simulink model "VELO1"  (R2019b)
settings: Solver=FixedStepAuto  StartTime=0.0  StopTime=t(end)  FixedStep=0.01  RelTol=1e-3
libraries: eeGeneralControl x26, dspstat3 x15, dspfdesign x11, sharedTrackingLibrary x2
(part 2 of 2)

== matlab function VELO1/Raw data filer /Subsystem2/MATLAB Function ==
  data: z1 input; x_hat output; z2 input; z3 input
function x_hat=fusion(z1,z2,z3)
% Kalman Filter sensor fusion example based on
%  
% http://www.slideshare.net/antoniomorancardenas/data-fusion-with-kalman-filtering
%
% % See http://home.wlu.edu/~levys/kalman_tutorial for background

% Copyright (C) 2014 Simon D. Levy
%
% This code is free software: you can redistribute it and/or modify
% it under the terms of the GNU Lesser General Public License as
% published by the Free Software Foundation, either version 3 of the
% License, or (at your option) any later version.
%
% This code is distributed in the hope that it will be useful,
% but WITHOUT ANY WARRANTY without even the implied warranty of
% MERCHANTABILITY or FITNESS FOR A PARTICULAR PURPOSE. See the
% GNU General Public License for more details.
%
% You should have received a copy of the GNU Lesser General Public License
% along with this code. If not, see <http:#www.gnu.org/licenses/>.

% Parameters ============================================================

% Biases
% BIAS1 = +1;
% BIAS2 = -1;

% Measurement noise covariances
R1 = 0.64;
R2 = 0.64;
R3 = 0.64;
% Process noise covariance
Q = .005;

% State transition model
A = 1;

% Observation model
C1 = 1;
C2 = 1;
C3=1;
% Duration
% N = 1000;

% Run ====================================================================

% Generate the signal x as a sine wave
% x = 20 + sin(5*linspace(0,1,N)*pi);

% Add some process noise with covariance Q
% w = sqrt(Q) * randn(size(x));
% x = x + w;

% Compute noisy sensor values
% z1 = BIAS1 + x + sqrt(R1) * randn(size(x));
% z2 = BIAS2 + x + sqrt(R2) * randn(size(x));

% Run a single-sensor example and plot it
% xhat = kalman(z1, A, C1, R1, Q);
% 
% % Plot sensed and estimated values
% clf
% plotsigs(1, z1, xhat, 'Sensor 1')
% title('One sensor: signal cleanup')
% 
% % Plot estimate and actual values
% plotsigsrms('One sensor', 2, x, xhat)

% Run the Kalman filter on fused sensors
x_hat = kalman([z1; z2; z3], A, [C1; C2 ;C3], [R1 0 0; 0 R2 0;0 0 R3], [Q;Q;Q]);
end

% Plot fusion example


% Helper functions ======================================================

== matlab function VELO1/Raw data filer /Subsystem3/MATLAB Function ==
  data: z1 input; x_hat output; z2 input; z3 input
function x_hat=fusion(z1,z2,z3)
% Kalman Filter sensor fusion example based on
%  
% http://www.slideshare.net/antoniomorancardenas/data-fusion-with-kalman-filtering
%
% % See http://home.wlu.edu/~levys/kalman_tutorial for background

% Copyright (C) 2014 Simon D. Levy
%
% This code is free software: you can redistribute it and/or modify
% it under the terms of the GNU Lesser General Public License as
% published by the Free Software Foundation, either version 3 of the
% License, or (at your option) any later version.
%
% This code is distributed in the hope that it will be useful,
% but WITHOUT ANY WARRANTY without even the implied warranty of
% MERCHANTABILITY or FITNESS FOR A PARTICULAR PURPOSE. See the
% GNU General Public License for more details.
%
% You should have received a copy of the GNU Lesser General Public License
% along with this code. If not, see <http:#www.gnu.org/licenses/>.

% Parameters ============================================================

% Biases
% BIAS1 = +1;
% BIAS2 = -1;

% Measurement noise covariances
R1 = 0.64;
R2 = 0.64;
R3 = 0.64;
% Process noise covariance
Q = .005;

% State transition model
A = 1;

% Observation model
C1 = 1;
C2 = 1;
C3=1;
% Duration
% N = 1000;

% Run ====================================================================

% Generate the signal x as a sine wave
% x = 20 + sin(5*linspace(0,1,N)*pi);

% Add some process noise with covariance Q
% w = sqrt(Q) * randn(size(x));
% x = x + w;

% Compute noisy sensor values
% z1 = BIAS1 + x + sqrt(R1) * randn(size(x));
% z2 = BIAS2 + x + sqrt(R2) * randn(size(x));

% Run a single-sensor example and plot it
% xhat = kalman(z1, A, C1, R1, Q);
% 
% % Plot sensed and estimated values
% clf
% plotsigs(1, z1, xhat, 'Sensor 1')
% title('One sensor: signal cleanup')
% 
% % Plot estimate and actual values
% plotsigsrms('One sensor', 2, x, xhat)

% Run the Kalman filter on fused sensors
x_hat = kalman([z1; z2; z3], A, [C1; C2 ;C3], [R1 0 0; 0 R2 0;0 0 R3], [Q;Q;Q]);
end

% Plot fusion example


% Helper functions ======================================================

== matlab function VELO1/Raw data filer /Subsystem4/MATLAB Function ==
  data: z1 input; x_hat output; z2 input; z3 input
function x_hat=fusion(z1,z2,z3)
% Kalman Filter sensor fusion example based on
%  
% http://www.slideshare.net/antoniomorancardenas/data-fusion-with-kalman-filtering
%
% % See http://home.wlu.edu/~levys/kalman_tutorial for background

% Copyright (C) 2014 Simon D. Levy
%
% This code is free software: you can redistribute it and/or modify
% it under the terms of the GNU Lesser General Public License as
% published by the Free Software Foundation, either version 3 of the
% License, or (at your option) any later version.
%
% This code is distributed in the hope that it will be useful,
% but WITHOUT ANY WARRANTY without even the implied warranty of
% MERCHANTABILITY or FITNESS FOR A PARTICULAR PURPOSE. See the
% GNU General Public License for more details.
%
% You should have received a copy of the GNU Lesser General Public License
% along with this code. If not, see <http:#www.gnu.org/licenses/>.

% Parameters ============================================================

% Biases
% BIAS1 = +1;
% BIAS2 = -1;

% Measurement noise covariances
R1 = 0.64;
R2 = 0.64;
R3 = 0.64;
% Process noise covariance
Q = .005;

% State transition model
A = 1;

% Observation model
C1 = 1;
C2 = 1;
C3=1;
% Duration
% N = 1000;

% Run ====================================================================

% Generate the signal x as a sine wave
% x = 20 + sin(5*linspace(0,1,N)*pi);

% Add some process noise with covariance Q
% w = sqrt(Q) * randn(size(x));
% x = x + w;

% Compute noisy sensor values
% z1 = BIAS1 + x + sqrt(R1) * randn(size(x));
% z2 = BIAS2 + x + sqrt(R2) * randn(size(x));

% Run a single-sensor example and plot it
% xhat = kalman(z1, A, C1, R1, Q);
% 
% % Plot sensed and estimated values
% clf
% plotsigs(1, z1, xhat, 'Sensor 1')
% title('One sensor: signal cleanup')
% 
% % Plot estimate and actual values
% plotsigsrms('One sensor', 2, x, xhat)

% Run the Kalman filter on fused sensors
x_hat = kalman([z1; z2; z3], A, [C1; C2 ;C3], [R1 0 0; 0 R2 0;0 0 R3], [Q;Q;Q]);
end

% Plot fusion example


% Helper functions ======================================================

== matlab function VELO1/Raw data filer /Subsystem5/MATLAB Function ==
  data: z1 input; x_hat output; z2 input; z3 input
function x_hat=fusion(z1,z2,z3)
% Kalman Filter sensor fusion example based on
%  
% http://www.slideshare.net/antoniomorancardenas/data-fusion-with-kalman-filtering
%
% % See http://home.wlu.edu/~levys/kalman_tutorial for background

% Copyright (C) 2014 Simon D. Levy
%
% This code is free software: you can redistribute it and/or modify
% it under the terms of the GNU Lesser General Public License as
% published by the Free Software Foundation, either version 3 of the
% License, or (at your option) any later version.
%
% This code is distributed in the hope that it will be useful,
% but WITHOUT ANY WARRANTY without even the implied warranty of
% MERCHANTABILITY or FITNESS FOR A PARTICULAR PURPOSE. See the
% GNU General Public License for more details.
%
% You should have received a copy of the GNU Lesser General Public License
% along with this code. If not, see <http:#www.gnu.org/licenses/>.

% Parameters ============================================================

% Biases
% BIAS1 = +1;
% BIAS2 = -1;

% Measurement noise covariances
R1 = 0.64;
R2 = 0.64;
R3 = 0.64;
% Process noise covariance
Q = .005;

% State transition model
A = 1;

% Observation model
C1 = 1;
C2 = 1;
C3=1;
% Duration
% N = 1000;

% Run ====================================================================

% Generate the signal x as a sine wave
% x = 20 + sin(5*linspace(0,1,N)*pi);

% Add some process noise with covariance Q
% w = sqrt(Q) * randn(size(x));
% x = x + w;

% Compute noisy sensor values
% z1 = BIAS1 + x + sqrt(R1) * randn(size(x));
% z2 = BIAS2 + x + sqrt(R2) * randn(size(x));

% Run a single-sensor example and plot it
% xhat = kalman(z1, A, C1, R1, Q);
% 
% % Plot sensed and estimated values
% clf
% plotsigs(1, z1, xhat, 'Sensor 1')
% title('One sensor: signal cleanup')
% 
% % Plot estimate and actual values
% plotsigsrms('One sensor', 2, x, xhat)

% Run the Kalman filter on fused sensors
x_hat = kalman([z1; z2; z3], A, [C1; C2 ;C3], [R1 0 0; 0 R2 0;0 0 R3], [Q;Q;Q]);
end

% Plot fusion example


% Helper functions ======================================================

== matlab function VELO1/Raw data filer /Subsystem6/MATLAB Function ==
  data: z1 input; x_hat output; z2 input; z3 input
function x_hat=fusion(z1,z2,z3)
% Kalman Filter sensor fusion example based on
%  
% http://www.slideshare.net/antoniomorancardenas/data-fusion-with-kalman-filtering
%
% % See http://home.wlu.edu/~levys/kalman_tutorial for background

% Copyright (C) 2014 Simon D. Levy
%
% This code is free software: you can redistribute it and/or modify
% it under the terms of the GNU Lesser General Public License as
% published by the Free Software Foundation, either version 3 of the
% License, or (at your option) any later version.
%
% This code is distributed in the hope that it will be useful,
% but WITHOUT ANY WARRANTY without even the implied warranty of
% MERCHANTABILITY or FITNESS FOR A PARTICULAR PURPOSE. See the
% GNU General Public License for more details.
%
% You should have received a copy of the GNU Lesser General Public License
% along with this code. If not, see <http:#www.gnu.org/licenses/>.

% Parameters ============================================================

% Biases
% BIAS1 = +1;
% BIAS2 = -1;

% Measurement noise covariances
R1 = 0.64;
R2 = 0.64;
R3 = 0.64;
% Process noise covariance
Q = .005;

% State transition model
A = 1;

% Observation model
C1 = 1;
C2 = 1;
C3=1;
% Duration
% N = 1000;

% Run ====================================================================

% Generate the signal x as a sine wave
% x = 20 + sin(5*linspace(0,1,N)*pi);

% Add some process noise with covariance Q
% w = sqrt(Q) * randn(size(x));
% x = x + w;

% Compute noisy sensor values
% z1 = BIAS1 + x + sqrt(R1) * randn(size(x));
% z2 = BIAS2 + x + sqrt(R2) * randn(size(x));

% Run a single-sensor example and plot it
% xhat = kalman(z1, A, C1, R1, Q);
% 
% % Plot sensed and estimated values
% clf
% plotsigs(1, z1, xhat, 'Sensor 1')
% title('One sensor: signal cleanup')
% 
% % Plot estimate and actual values
% plotsigsrms('One sensor', 2, x, xhat)

% Run the Kalman filter on fused sensors
x_hat = kalman([z1; z2; z3], A, [C1; C2 ;C3], [R1 0 0; 0 R2 0;0 0 R3], [Q;Q;Q]);
end

% Plot fusion example


% Helper functions ======================================================

== matlab function VELO1/Subsystem3/MATLAB Function ==
  data: z1 input; x_hat output; z2 input; z3 input
function x_hat=fusion(z1,z2,z3)
% Kalman Filter sensor fusion example based on
%  
% http://www.slideshare.net/antoniomorancardenas/data-fusion-with-kalman-filtering
%
% % See http://home.wlu.edu/~levys/kalman_tutorial for background

% Copyright (C) 2014 Simon D. Levy
%
% This code is free software: you can redistribute it and/or modify
% it under the terms of the GNU Lesser General Public License as
% published by the Free Software Foundation, either version 3 of the
% License, or (at your option) any later version.
%
% This code is distributed in the hope that it will be useful,
% but WITHOUT ANY WARRANTY without even the implied warranty of
% MERCHANTABILITY or FITNESS FOR A PARTICULAR PURPOSE. See the
% GNU General Public License for more details.
%
% You should have received a copy of the GNU Lesser General Public License
% along with this code. If not, see <http:#www.gnu.org/licenses/>.

% Parameters ============================================================

% Biases
% BIAS1 = +1;
% BIAS2 = -1;

% Measurement noise covariances
R1 = 0.1;
R2 = 0.7;
R3 = 0.1;
% Process noise covariance
Q = .005;

% State transition model
A = 1;

% Observation model
C1 = 1;
C2 = 1;
C3=1;
% Duration
% N = 1000;

% Run ====================================================================

% Generate the signal x as a sine wave
% x = 20 + sin(5*linspace(0,1,N)*pi);

% Add some process noise with covariance Q
% w = sqrt(Q) * randn(size(x));
% x = x + w;

% Compute noisy sensor values
% z1 = BIAS1 + x + sqrt(R1) * randn(size(x));
% z2 = BIAS2 + x + sqrt(R2) * randn(size(x));

% Run a single-sensor example and plot it
% xhat = kalman(z1, A, C1, R1, Q);
% 
% % Plot sensed and estimated values
% clf
% plotsigs(1, z1, xhat, 'Sensor 1')
% title('One sensor: signal cleanup')
% 
% % Plot estimate and actual values
% plotsigsrms('One sensor', 2, x, xhat)

% Run the Kalman filter on fused sensors
x_hat = kalman([z1; z2; z3], A, [C1; C2 ;C3], [R1 0 0; 0 R2 0;0 0 R3], [Q;Q;Q]);
end

% Plot fusion example


% Helper functions ======================================================

== matlab function VELO1/speed/MATLAB Function1 ==
  data: z1 input; x_hat output; z2 input; z3 input
function x_hat=fusion(z1,z2,z3)
% Kalman Filter sensor fusion example based on
%  
% http://www.slideshare.net/antoniomorancardenas/data-fusion-with-kalman-filtering
%
% % See http://home.wlu.edu/~levys/kalman_tutorial for background

% Copyright (C) 2014 Simon D. Levy
%
% This code is free software: you can redistribute it and/or modify
% it under the terms of the GNU Lesser General Public License as
% published by the Free Software Foundation, either version 3 of the
% License, or (at your option) any later version.
%
% This code is distributed in the hope that it will be useful,
% but WITHOUT ANY WARRANTY without even the implied warranty of
% MERCHANTABILITY or FITNESS FOR A PARTICULAR PURPOSE. See the
% GNU General Public License for more details.
%
% You should have received a copy of the GNU Lesser General Public License
% along with this code. If not, see <http:#www.gnu.org/licenses/>.

% Parameters ============================================================

% Biases
% BIAS1 = +1;
% BIAS2 = -1;

% Measurement noise covariances
R1 = 0.64;
R2 = 0.64;
R3 = 0.64;
% Process noise covariance
Q = .005;

% State transition model
A = 1;

% Observation model
C1 = 1;
C2 = 1;
C3=1;
% Duration
% N = 1000;

% Run ====================================================================

% Generate the signal x as a sine wave
% x = 20 + sin(5*linspace(0,1,N)*pi);

% Add some process noise with covariance Q
% w = sqrt(Q) * randn(size(x));
% x = x + w;

% Compute noisy sensor values
% z1 = BIAS1 + x + sqrt(R1) * randn(size(x));
% z2 = BIAS2 + x + sqrt(R2) * randn(size(x));

% Run a single-sensor example and plot it
% xhat = kalman(z1, A, C1, R1, Q);
% 
% % Plot sensed and estimated values
% clf
% plotsigs(1, z1, xhat, 'Sensor 1')
% title('One sensor: signal cleanup')
% 
% % Plot estimate and actual values
% plotsigsrms('One sensor', 2, x, xhat)

% Run the Kalman filter on fused sensors
x_hat = kalman([z1; z2; z3], A, [C1; C2 ;C3], [R1 0 0; 0 R2 0;0 0 R3], [Q;Q;Q]);
end

% Plot fusion example


% Helper functions ======================================================

== matlab function VELO1/pitch roll yaw dispacement/MATLAB Function1 ==
  data: v_w input; s output; v_v input
function s = fcn(v_w,v_v)

s =100* (v_w-v_v)/max(v_w,v_v);
end

== matlab function VELO1/Subsystem1/MATLAB Function ==
  data: ax input; a output; ay input; az input
function a = fcn(ax,ay,az)
a=sqrt(ax^2+ay^2+az^2);
end

== matlab function VELO1/MATLAB Function ==
  data: ax input; teta0 output; az input; ay input; phi0 output
function [teta0,phi0] = fcn(ax,az,ay)

teta0=atan(ax/az);
phi0=atan(ay/az);

end

== matlab function VELO1/Raw data filer /MATLAB Function1 ==
  data: ax input; az_pp output; ay input; az input; ax_pp output; ay_pp output; teta0 input; phi0 input; psi0 input; a_abs input
function [az_pp,ax_pp,ay_pp] = fcn(ax,ay,az,teta0,phi0,psi0,a_abs)
gain=1/a_abs;

az_p=az*cos(teta0)+ax*sin(teta0);
ax_p=ax*cos(teta0)-az*sin(teta0);

az_pp=gain*(az_p*cos(phi0)+ay*sin(phi0));
ay_p=ay*cos(phi0)-az_p*sin(phi0);
ax_pp=gain*(ax_p*cos(psi0)+ay_p*sin(psi0));
ay_pp=gain*(ay_p*cos(psi0)-ax_p*sin(psi0));
end

== matlab function VELO1/Raw data filer /MATLAB Function2 ==
  data: ax input; az_pp output; ay input; az input; ax_pp output; ay_pp output; teta0 input; phi0 input; psi0 input; a_abs input
function [az_pp,ax_pp,ay_pp] = fcn(ax,ay,az,teta0,phi0,psi0,a_abs)
gain=1/a_abs;

az_p=az*cos(teta0)+ax*sin(teta0);
ax_p=ax*cos(teta0)-az*sin(teta0);

az_pp=gain*(az_p*cos(phi0)+ay*sin(phi0));
ay_p=ay*cos(phi0)-az_p*sin(phi0);
ax_pp=gain*(ax_p*cos(psi0)+ay_p*sin(psi0));
ay_pp=gain*(ay_p*cos(psi0)-ax_p*sin(psi0));
end

== matlab function VELO1/MATLAB Function2 ==
  data: accz input; grade output
function grade = fcn(accz)

grade=(400/pi)*acos(accz/1);
end

== matlab function VELO1/MATLAB Function1 ==
  data: graden input; ay input; ax input; az input; grade0 input; grade output; flag output
function [grade,flag] = fcn(graden,ay,ax,az,grade0)
if abs(ay)<=0.051&& abs(ax)<=0.051 && abs(az)<=1
    grade=graden;
    flag=1;
else
    grade=grade0;
flag=0;
end

end

== matlab function VELO1/Longitudinal Force Est./MATLAB Function ==
  data: Ax input; Fx output; Vx input; m input
function Fx = fcn(Ax, Vx, m)

g = 9.81;

Da = 0.4; % Aerodynamics overall coefficient
fR = 0.02; % Rolling resistance coefficient
Fr = fR*m*g;

if Ax >= 0
    
    Fx = m*abs(Ax) + abs(Fr) + abs(Da*Vx^2);
    
else
    
    Fx = (m*abs(Ax) - abs(Fr) - abs(Da*Vx^2)) / 2; % When braking, both front and rear axles are engaged

end

== matlab function VELO1/Longitudinal Force Est./MATLAB Function1 ==
  data: Ax input; Fx output; Vx input; m input
function Fx = fcn(Ax, Vx, m)

g = 9.81;

Da = 0.4; % Aerodynamics overall coefficient
fR = 0.02; % Rolling resistance coefficient
Fr = fR*m*g;

if Ax >= 0
    
    Fx = m*abs(Ax) + abs(Fr) + abs(Da*Vx^2);
    
else
    
    Fx = (m*abs(Ax) - abs(Fr) - abs(Da*Vx^2)) / 2; % When braking, both front and rear axles are engaged
        
end

== matlab function VELO1/Normal Force Est./MATLAB Function ==
  data: Ax input; Fzf output; Vx input; m input; Fzr output
function [Fzf, Fzr] = fcn(Ax, Vx, m)

g = 9.81;
Lf = 1/4 * 1.7;
Lr = 3/4 * 1.7;
h = 0.4;
ha = 0.5;

Da = 0.4; % Aerodynamics overall coefficient
L = Lf + Lr;
    
Fzf = (m*g*Lr - m*Ax*h - ha*Da*Vx^2)/L;
    
Fzr = (m*g*Lf + m*Ax*h + ha*Da*Vx^2)/L;
        
end

== matlab function VELO1/Normal Force Est./MATLAB Function1 ==
  data: Ax input; Fzf output; Vx input; m input; Fzr output
function [Fzf, Fzr] = fcn(Ax, Vx, m)

g = 9.81;
Lf = 1/4 * 1.7;
Lr = 3/4 * 1.7;
h = 0.4;
ha = 0.5;

Da = 0.4; % Aerodynamics overall coefficient
L = Lf + Lr;
    
Fzf = (m*g*Lr - m*Ax*h - ha*Da*Vx^2)/L;
    
Fzr = (m*g*Lf + m*Ax*h + ha*Da*Vx^2)/L;
        
end
